simulink model "FDIBenchMark_BLW_66_71"  (Simulink 6.3)
settings: Solver=ode45  StartTime=0.0  StopTime=300  FixedStep=Ts  RelTol=1e-12
InitFcn:
  | FDIBenchMarkData
undefined symbols (not defined in the file or in its folder): a, Addt, Addt2, alpha, alpha_gc, Apb, Apb1, Apb2, Bddt, Bddt2, Bpb, Bpb1, Bpb2, Cddt, Constant_Beta_1_m1, Constant_Beta_3_m1, Constant_Omega_r_m1, Constant_tau_gc, Cpb, Cpb1, Cpb2, Cq, DiscIntNeverNeededParam, eta_gc, Gain_Beta_2_m2, Gain_Omega_r_m2, H, k, K_opt, L, m, m_vw, Omega_delta, omega_n, Omega_nom, P_r, R, r, r0, rho, seed, T_sample, Ts, turb_int, turbulence_seeds, u0, xi
libraries: simulink x13
(part 2 of 2)

== matlab function Controller/Embedded MATLAB Function ==
  data: P_g input double; ControlZone output double; P_r input double; Omega_g input double; LastControlZone input double; Omega_nom input double; Omega_delta input double
function ControlZone = ZoneControl(P_g, P_r, Omega_g, LastControlZone,Omega_nom,Omega_delta)
 
if LastControlZone==0,
    if (P_g>=P_r) ||(Omega_g>=Omega_nom)
        ControlZone=1;
    else
        ControlZone=0;
    end
else
    if (Omega_g<(Omega_nom-Omega_delta))
        ControlZone=0;
    else
        ControlZone=1;
    end
end
